simulink model "TestbedModel_v6"  (R2016a)
settings: Solver=ode23tb  StartTime=0.0  StopTime=20  RelTol=1e-3
undefined symbols (not defined in the file): K, Ki, Kp, magnitude, rev_comms_sink, tau
libraries: DAEMOT_Lib x4
(part 4 of 4)

== system TestbedModel_v6/Bus/Sink1 ==
  In1 : Inport
  tag scope: gdata_TestbedModel_v6BusSink1=global
  wires:
  In1/1 -> [gdata_TestbedModel_v6BusSink1]

== system TestbedModel_v6/Bus/Source1 ==
  Out1 : Outport
  wires:
  [gdata_TestbedModel_v6EffortSink9Sink1] -> Out1/1

== system TestbedModel_v6/Bus/Source2 ==
  Out1 : Outport
  wires:
  [gdata_TestbedModel_v6Converter2Sink1] -> Out1/1

== system TestbedModel_v6/Capacitor/Data_Sink ==
  " " : Inport
  tag scope: gdata_CapacitorData_Sink=global
  wires:
  " "/1 -> [gdata_CapacitorData_Sink]

== system TestbedModel_v6/Capacitor/Sink1 ==
  In1 : Inport
  tag scope: gdata_TestbedModel_v6CapacitorSink1=global
  wires:
  In1/1 -> [gdata_TestbedModel_v6CapacitorSink1]

== system TestbedModel_v6/Capacitor/Source1 ==
  Out1 : Outport
  wires:
  [gdata_TestbedModel_v6ResistorSink1] -> Out1/1

== system TestbedModel_v6/Capacitor1/Data_Sink ==
  " " : Inport
  tag scope: gdata_Capacitor1Data_Sink=global
  wires:
  " "/1 -> [gdata_Capacitor1Data_Sink]

== system TestbedModel_v6/Capacitor1/Sink1 ==
  In1 : Inport
  tag scope: gdata_TestbedModel_v6Capacitor1Sink1=global
  wires:
  In1/1 -> [gdata_TestbedModel_v6Capacitor1Sink1]

== system TestbedModel_v6/Capacitor1/Source1 ==
  Out1 : Outport
  wires:
  [gdata_TestbedModel_v6EffortSink13Sink1] -> Out1/1

== system TestbedModel_v6/Converter/Data_Sink ==
  " " : Inport
  tag scope: gdata_ConverterData_Sink=global
  wires:
  " "/1 -> [gdata_ConverterData_Sink]

== system TestbedModel_v6/Converter/Sink1 ==
  In1 : Inport
  tag scope: gdata_TestbedModel_v6ConverterSink1=global
  wires:
  In1/1 -> [gdata_TestbedModel_v6ConverterSink1]

== system TestbedModel_v6/Converter/Source1 ==
  Out1 : Outport
  wires:
  [gdata_TestbedModel_v6MotorSink1] -> Out1/1

== system TestbedModel_v6/Converter/Source2 ==
  Out1 : Outport
  wires:
  [gdata_TestbedModel_v6EffortSink2Sink1] -> Out1/1

== system TestbedModel_v6/Converter1/Data_Sink ==
  " " : Inport
  tag scope: gdata_Converter1Data_Sink=global
  wires:
  " "/1 -> [gdata_Converter1Data_Sink]

== system TestbedModel_v6/Converter1/Sink1 ==
  In1 : Inport
  tag scope: gdata_TestbedModel_v6Converter1Sink1=global
  wires:
  In1/1 -> [gdata_TestbedModel_v6Converter1Sink1]

== system TestbedModel_v6/Converter1/Source1 ==
  Out1 : Outport
  wires:
  [gdata_TestbedModel_v6InductorSink1] -> Out1/1

== system TestbedModel_v6/Converter1/Source2 ==
  Out1 : Outport
  wires:
  [gdata_TestbedModel_v6EffortSink5Sink1] -> Out1/1

== system TestbedModel_v6/Converter2/Data_Sink ==
  " " : Inport
  tag scope: gdata_Converter2Data_Sink=global
  wires:
  " "/1 -> [gdata_Converter2Data_Sink]

== system TestbedModel_v6/Converter2/Sink1 ==
  In1 : Inport
  tag scope: gdata_TestbedModel_v6Converter2Sink1=global
  wires:
  In1/1 -> [gdata_TestbedModel_v6Converter2Sink1]

== system TestbedModel_v6/Converter2/Source1 ==
  Out1 : Outport
  wires:
  [gdata_TestbedModel_v6Motor1Sink1] -> Out1/1

== system TestbedModel_v6/Converter2/Source2 ==
  Out1 : Outport
  wires:
  [gdata_TestbedModel_v6EffortSink8Sink1] -> Out1/1

== system TestbedModel_v6/Converter3/Data_Sink ==
  " " : Inport
  tag scope: gdata_Converter3Data_Sink=global
  wires:
  " "/1 -> [gdata_Converter3Data_Sink]

== system TestbedModel_v6/Converter3/Sink1 ==
  In1 : Inport
  tag scope: gdata_TestbedModel_v6Converter3Sink1=global
  wires:
  In1/1 -> [gdata_TestbedModel_v6Converter3Sink1]

== system TestbedModel_v6/Converter3/Source1 ==
  Out1 : Outport
  wires:
  [gdata_TestbedModel_v6Inductor1Sink1] -> Out1/1

== system TestbedModel_v6/Converter3/Source2 ==
  Out1 : Outport
  wires:
  [gdata_TestbedModel_v6EffortSink11Sink1] -> Out1/1

== system TestbedModel_v6/Data Manager/SubSystem1 ==
  Rename : Inport
  Bus : Outport
  wires:
  Rename/1 -> Bus/1

== system TestbedModel_v6/Data Manager1/SubSystem1 ==
  Rename : Inport
  Bus : Outport
  wires:
  Rename/1 -> Bus/1

== system TestbedModel_v6/Data Manager10/SubSystem1 ==
  Rename : Inport
  Bus : Outport
  wires:
  Rename/1 -> Bus/1

== system TestbedModel_v6/Data Manager11/SubSystem1 ==
  Rename : Inport
  Bus : Outport
  wires:
  Rename/1 -> Bus/1

== system TestbedModel_v6/Data Manager12/SubSystem1 ==
  Rename : Inport
  Bus : Outport
  wires:
  Rename/1 -> Bus/1

== system TestbedModel_v6/Data Manager13/SubSystem1 ==
  Rename : Inport
  Bus : Outport
  wires:
  Rename/1 -> Bus/1

== system TestbedModel_v6/Data Manager14/SubSystem1 ==
  Rename : Inport
  Bus : Outport
  wires:
  Rename/1 -> Bus/1

== system TestbedModel_v6/Data Manager15/SubSystem1 ==
  Rename : Inport
  Bus : Outport
  wires:
  Rename/1 -> Bus/1

== system TestbedModel_v6/Data Manager15/SubSystem2 ==
  Rename : Inport
  Bus : Outport
  wires:
  Rename/1 -> Bus/1

== system TestbedModel_v6/Data Manager16/SubSystem1 ==
  Rename : Inport
  Bus : Outport
  wires:
  Rename/1 -> Bus/1

== system TestbedModel_v6/Data Manager16/SubSystem2 ==
  Rename : Inport
  Bus : Outport
  wires:
  Rename/1 -> Bus/1

== system TestbedModel_v6/Data Manager16/SubSystem3 ==
  Rename : Inport
  Bus : Outport
  wires:
  Rename/1 -> Bus/1

== system TestbedModel_v6/Data Manager16/SubSystem4 ==
  Rename : Inport
  Bus : Outport
  wires:
  Rename/1 -> Bus/1

== system TestbedModel_v6/Data Manager17/SubSystem1 ==
  Rename : Inport
  Bus : Outport
  wires:
  Rename/1 -> Bus/1

== system TestbedModel_v6/Data Manager18/SubSystem1 ==
  Rename : Inport
  Bus : Outport
  wires:
  Rename/1 -> Bus/1

== system TestbedModel_v6/Data Manager19/SubSystem1 ==
  Rename : Inport
  Bus : Outport
  wires:
  Rename/1 -> Bus/1

== system TestbedModel_v6/Data Manager19/SubSystem2 ==
  Rename : Inport
  Bus : Outport
  wires:
  Rename/1 -> Bus/1

== system TestbedModel_v6/Data Manager2/SubSystem1 ==
  Rename : Inport
  Bus : Outport
  wires:
  Rename/1 -> Bus/1

== system TestbedModel_v6/Data Manager20/SubSystem1 ==
  Rename : Inport
  Bus : Outport
  wires:
  Rename/1 -> Bus/1

== system TestbedModel_v6/Data Manager21/SubSystem1 ==
  Rename : Inport
  Bus : Outport
  wires:
  Rename/1 -> Bus/1

== system TestbedModel_v6/Data Manager22/SubSystem1 ==
  Rename : Inport
  Bus : Outport
  wires:
  Rename/1 -> Bus/1

== system TestbedModel_v6/Data Manager23/SubSystem1 ==
  Rename : Inport
  Bus : Outport
  wires:
  Rename/1 -> Bus/1

== system TestbedModel_v6/Data Manager24/SubSystem1 ==
  Rename : Inport
  Bus : Outport
  wires:
  Rename/1 -> Bus/1

== system TestbedModel_v6/Data Manager25/SubSystem1 ==
  Rename : Inport
  Bus : Outport
  wires:
  Rename/1 -> Bus/1

== system TestbedModel_v6/Data Manager3/SubSystem1 ==
  Rename : Inport
  Bus : Outport
  wires:
  Rename/1 -> Bus/1

== system TestbedModel_v6/Data Manager4/SubSystem1 ==
  Rename : Inport
  Bus : Outport
  wires:
  Rename/1 -> Bus/1

== system TestbedModel_v6/Data Manager5/SubSystem1 ==
  Rename : Inport
  Bus : Outport
  wires:
  Rename/1 -> Bus/1

== system TestbedModel_v6/Data Manager6/SubSystem1 ==
  Rename : Inport
  Bus : Outport
  wires:
  Rename/1 -> Bus/1

== system TestbedModel_v6/Data Manager6/SubSystem2 ==
  Rename : Inport
  Bus : Outport
  wires:
  Rename/1 -> Bus/1

== system TestbedModel_v6/Data Manager7/SubSystem1 ==
  Rename : Inport
  Bus : Outport
  wires:
  Rename/1 -> Bus/1

== system TestbedModel_v6/Data Manager8/SubSystem1 ==
  Rename : Inport
  Bus : Outport
  wires:
  Rename/1 -> Bus/1

== system TestbedModel_v6/Data Manager9/SubSystem1 ==
  Rename : Inport
  Bus : Outport
  wires:
  Rename/1 -> Bus/1

== system TestbedModel_v6/Effort Sink1/Sink1 ==
  In1 : Inport
  tag scope: gdata_TestbedModel_v6EffortSink1Sink1=global
  wires:
  In1/1 -> [gdata_TestbedModel_v6EffortSink1Sink1]

== system TestbedModel_v6/Effort Sink10/Sink1 ==
  In1 : Inport
  tag scope: gdata_TestbedModel_v6EffortSink10Sink1=global
  wires:
  In1/1 -> [gdata_TestbedModel_v6EffortSink10Sink1]

== system TestbedModel_v6/Effort Sink11/Sink1 ==
  In1 : Inport
  tag scope: gdata_TestbedModel_v6EffortSink11Sink1=global
  wires:
  In1/1 -> [gdata_TestbedModel_v6EffortSink11Sink1]

== system TestbedModel_v6/Effort Sink12/Sink1 ==
  In1 : Inport
  tag scope: gdata_TestbedModel_v6EffortSink12Sink1=global
  wires:
  In1/1 -> [gdata_TestbedModel_v6EffortSink12Sink1]

== system TestbedModel_v6/Effort Sink13/Sink1 ==
  In1 : Inport
  tag scope: gdata_TestbedModel_v6EffortSink13Sink1=global
  wires:
  In1/1 -> [gdata_TestbedModel_v6EffortSink13Sink1]

== system TestbedModel_v6/Effort Sink14/Sink1 ==
  In1 : Inport
  tag scope: gdata_TestbedModel_v6EffortSink14Sink1=global
  wires:
  In1/1 -> [gdata_TestbedModel_v6EffortSink14Sink1]

== system TestbedModel_v6/Effort Sink15/Sink1 ==
  In1 : Inport
  tag scope: gdata_TestbedModel_v6EffortSink15Sink1=global
  wires:
  In1/1 -> [gdata_TestbedModel_v6EffortSink15Sink1]

== system TestbedModel_v6/Effort Sink16/Sink1 ==
  In1 : Inport
  tag scope: gdata_TestbedModel_v6EffortSink16Sink1=global
  wires:
  In1/1 -> [gdata_TestbedModel_v6EffortSink16Sink1]

== system TestbedModel_v6/Effort Sink2/Sink1 ==
  In1 : Inport
  tag scope: gdata_TestbedModel_v6EffortSink2Sink1=global
  wires:
  In1/1 -> [gdata_TestbedModel_v6EffortSink2Sink1]

== system TestbedModel_v6/Effort Sink3/Sink1 ==
  In1 : Inport
  tag scope: gdata_TestbedModel_v6EffortSink3Sink1=global
  wires:
  In1/1 -> [gdata_TestbedModel_v6EffortSink3Sink1]

== system TestbedModel_v6/Effort Sink4/Sink1 ==
  In1 : Inport
  tag scope: gdata_TestbedModel_v6EffortSink4Sink1=global
  wires:
  In1/1 -> [gdata_TestbedModel_v6EffortSink4Sink1]

== system TestbedModel_v6/Effort Sink5/Sink1 ==
  In1 : Inport
  tag scope: gdata_TestbedModel_v6EffortSink5Sink1=global
  wires:
  In1/1 -> [gdata_TestbedModel_v6EffortSink5Sink1]

== system TestbedModel_v6/Effort Sink6/Sink1 ==
  In1 : Inport
  tag scope: gdata_TestbedModel_v6EffortSink6Sink1=global
  wires:
  In1/1 -> [gdata_TestbedModel_v6EffortSink6Sink1]

== system TestbedModel_v6/Effort Sink7/Sink1 ==
  In1 : Inport
  tag scope: gdata_TestbedModel_v6EffortSink7Sink1=global
  wires:
  In1/1 -> [gdata_TestbedModel_v6EffortSink7Sink1]

== system TestbedModel_v6/Effort Sink8/Sink1 ==
  In1 : Inport
  tag scope: gdata_TestbedModel_v6EffortSink8Sink1=global
  wires:
  In1/1 -> [gdata_TestbedModel_v6EffortSink8Sink1]

== system TestbedModel_v6/Effort Sink9/Sink1 ==
  In1 : Inport
  tag scope: gdata_TestbedModel_v6EffortSink9Sink1=global
  wires:
  In1/1 -> [gdata_TestbedModel_v6EffortSink9Sink1]

== system TestbedModel_v6/Effort Source/Source1 ==
  Out1 : Outport
  wires:
  [gdata_TestbedModel_v6BatterySink1] -> Out1/1

== system TestbedModel_v6/Effort Source1/Source1 ==
  Out1 : Outport
  wires:
  [gdata_TestbedModel_v6VoltageBusSink1] -> Out1/1

== system TestbedModel_v6/Inductor/Data_Sink ==
  " " : Inport
  tag scope: gdata_InductorData_Sink=global
  wires:
  " "/1 -> [gdata_InductorData_Sink]

== system TestbedModel_v6/Inductor/Sink1 ==
  In1 : Inport
  tag scope: gdata_TestbedModel_v6InductorSink1=global
  wires:
  In1/1 -> [gdata_TestbedModel_v6InductorSink1]

== system TestbedModel_v6/Inductor/Source1 ==
  Out1 : Outport
  wires:
  [gdata_TestbedModel_v6CapacitorSink1] -> Out1/1

== system TestbedModel_v6/Inductor1/Data_Sink ==
  " " : Inport
  tag scope: gdata_Inductor1Data_Sink=global
  wires:
  " "/1 -> [gdata_Inductor1Data_Sink]

== system TestbedModel_v6/Inductor1/Sink1 ==
  In1 : Inport
  tag scope: gdata_TestbedModel_v6Inductor1Sink1=global
  wires:
  In1/1 -> [gdata_TestbedModel_v6Inductor1Sink1]

== system TestbedModel_v6/Inductor1/Source1 ==
  Out1 : Outport
  wires:
  [gdata_TestbedModel_v6Capacitor1Sink1] -> Out1/1

== system TestbedModel_v6/Motor/Data_Sink ==
  " " : Inport
  tag scope: gdata_MotorData_Sink=global
  wires:
  " "/1 -> [gdata_MotorData_Sink]

== system TestbedModel_v6/Motor/Sink1 ==
  In1 : Inport
  tag scope: gdata_TestbedModel_v6MotorSink1=global
  wires:
  In1/1 -> [gdata_TestbedModel_v6MotorSink1]

== system TestbedModel_v6/Motor/Source1 ==
  Out1 : Outport
  wires:
  [gdata_TestbedModel_v6EffortSink16Sink1] -> Out1/1

== system TestbedModel_v6/Motor/Source2 ==
  Out1 : Outport
  wires:
  [gdata_TestbedModel_v6EffortSink1Sink1] -> Out1/1

== system TestbedModel_v6/Motor1/Data_Sink ==
  " " : Inport
  tag scope: gdata_Motor1Data_Sink=global
  wires:
  " "/1 -> [gdata_Motor1Data_Sink]

== system TestbedModel_v6/Motor1/Sink1 ==
  In1 : Inport
  tag scope: gdata_TestbedModel_v6Motor1Sink1=global
  wires:
  In1/1 -> [gdata_TestbedModel_v6Motor1Sink1]

== system TestbedModel_v6/Motor1/Source1 ==
  Out1 : Outport
  wires:
  [gdata_TestbedModel_v6ShaftSink1] -> Out1/1

== system TestbedModel_v6/Motor1/Source2 ==
  Out1 : Outport
  wires:
  [gdata_TestbedModel_v6EffortSink7Sink1] -> Out1/1

== system TestbedModel_v6/Resistor/Data_Sink ==
  " " : Inport
  tag scope: gdata_ResistorData_Sink=global
  wires:
  " "/1 -> [gdata_ResistorData_Sink]

== system TestbedModel_v6/Resistor/Sink1 ==
  In1 : Inport
  tag scope: gdata_TestbedModel_v6ResistorSink1=global
  wires:
  In1/1 -> [gdata_TestbedModel_v6ResistorSink1]

== system TestbedModel_v6/Resistor/Source1 ==
  Out1 : Outport
  wires:
  [gdata_TestbedModel_v6EffortSink4Sink1] -> Out1/1

== system TestbedModel_v6/Resistor/Source2 ==
  Out1 : Outport
  wires:
  [gdata_TestbedModel_v6EffortSink3Sink1] -> Out1/1

== system TestbedModel_v6/Shaft/Data_Sink ==
  " " : Inport
  tag scope: gdata_ShaftData_Sink=global
  wires:
  " "/1 -> [gdata_ShaftData_Sink]

== system TestbedModel_v6/Shaft/Sink1 ==
  In1 : Inport
  tag scope: gdata_TestbedModel_v6ShaftSink1=global
  wires:
  In1/1 -> [gdata_TestbedModel_v6ShaftSink1]

== system TestbedModel_v6/Shaft/Source1 ==
  Out1 : Outport
  wires:
  [gdata_TestbedModel_v6AirVehicleSink1] -> Out1/1

== system TestbedModel_v6/Voltage Bus/Data_Sink ==
  " " : Inport
  tag scope: gdata_VoltageBusData_Sink=global
  wires:
  " "/1 -> [gdata_VoltageBusData_Sink]

== system TestbedModel_v6/Voltage Bus/Sink1 ==
  In1 : Inport
  tag scope: gdata_TestbedModel_v6VoltageBusSink1=global
  wires:
  In1/1 -> [gdata_TestbedModel_v6VoltageBusSink1]

== system TestbedModel_v6/Voltage Bus/Source1 ==
  Out1 : Outport
  wires:
  [gdata_TestbedModel_v6ConverterSink1] -> Out1/1

== system TestbedModel_v6/Voltage Bus/Source2 ==
  Out1 : Outport
  wires:
  [gdata_TestbedModel_v6Converter1Sink1] -> Out1/1

== matlab function TestbedModel_v6/Converter1/Current ==
  data: I_out input; D input; I_in output; s input; dir parameter
function I_in = current(I_out,D,s,dir)

if dir == 1 %Boost ===>
    if s == 0     % Buck Mode
        I_in = I_out/D;
    else    % Boost Mode
        I_in = I_out/(1-D);
    end
elseif dir == 2 %Boost <===
    if s == 0     % Buck Mode
        I_in = D*I_out;
    else    % Boost Mode
        I_in = (1-D)*I_out;
    end
end

== matlab function TestbedModel_v6/Converter1/Thermal ==
  data: Q input; T_dot output; Q_sink input; Cp parameter
function T_dot = Thermal(Q, Q_sink, Cp)
%% Load Temperature
T_dot = (1/Cp) * (Q - Q_sink);

== matlab function TestbedModel_v6/Converter1/Voltage ==
  data: V_in input; V_out output; I_in input; I_out input; D input; s input; V_D parameter; R_D parameter; R_s parameter; R_L parameter; Q output; dir parameter
function [V_out,Q]= voltage(V_in,I_in,I_out,D,s,V_D, R_D, R_s, R_L,dir)

if dir == 1 %Boost ===>
    I_L = I_in;
    if s == 0     % Buck Mode
        V_out = (1/D) * (V_in - R_L*I_L - D*R_s*I_L - (1-D)*R_D*I_L + (1-D)*V_D);
        Q = (1/D)^2 * (R_L*I_out^2 + D*R_s*I_out^2 + (1-D)*R_D*I_out^2);
    else    % Boost Mode
        V_out = (1/(1-D)) * (V_in - R_L*I_L - D*R_s*I_L - (1-D)*R_D*I_L - (1-D)*V_D);
        Q = (1/(1-D))^2 * (R_L*I_out^2 + D*R_s*I_out^2 + (1-D)*R_D*I_out^2);
    end
elseif dir == 2 %Boost <===
    I_L = I_out;
    if s == 0     % Buck Mode
        V_out = D*V_in - D*R_s*I_L - R_L*I_L - (1-D)*V_D - (1-D)*R_D*I_L;
        Q = (R_L*I_out^2 + D*R_s*I_out^2 + (1-D)*R_D*I_out^2);
    else    % Boost Mode
        V_out = (1-D)*V_in - D*R_s*I_L - R_L*I_L + (1-D)*V_D - (1-D)*R_D*I_L;
        Q = (R_L*I_out^2 + D*R_s*I_out^2 + (1-D)*R_D*I_out^2);
    end
end

== matlab function TestbedModel_v6/Inductor/Current ==
  data: V_in input; V_out input; dI_dt output; L parameter
function dI_dt = current(V_in, V_out,L)

dI_dt = (V_in-V_out)/L;

== matlab function TestbedModel_v6/Capacitor/Voltage ==
  data: I_in input; V_dot output; I_out input; C parameter
function V_dot = voltage(I_in, I_out,C)

V_dot = (1/C) * (I_in-I_out);

== matlab function TestbedModel_v6/Motor1/Current ==
  data: V_in input; I_in input; Kv parameter; R parameter; L parameter; omega input; dI_dt output; Q_elec output
function [dI_dt,Q_elec]= current(V_in,I_in,Kv, R, L,omega)


dI_dt = (1/L) * (V_in - R*I_in - Kv*omega);

Q_elec = R*I_in^2;

== matlab function TestbedModel_v6/Motor1/Thermal ==
  data: Q_elec input; Q_mech input; T_dot output; Q_sink input; Cp parameter
function T_dot = Thermal(Q_elec,Q_mech, Q_sink, Cp)
%% Load Temperature
T_dot = (1/Cp) * (Q_elec + Q_mech - Q_sink);

== matlab function TestbedModel_v6/Motor1/Torque ==
  data: I_in input; omega input; T_motor output; b parameter; c parameter; Q_mech output; Kv parameter
function [T_motor,Q_mech]= omega(I_in,omega, b,c,Kv)

T_motor = Kv*I_in - b*omega - c*(2./(1+exp(-5*omega)) - 1);

Q_mech = b*omega^2 + omega*(2./(1+exp(-5*omega)) - 1);

== matlab function TestbedModel_v6/Converter2/Current ==
  data: I_out input; D input; I_in output; s input; dir parameter
function I_in = current(I_out,D,s,dir)

if dir == 1 %Boost ===>
    if s == 0     % Buck Mode
        I_in = I_out/D;
    else    % Boost Mode
        I_in = I_out/(1-D);
    end
elseif dir == 2 %Boost <===
    if s == 0     % Buck Mode
        I_in = D*I_out;
    else    % Boost Mode
        I_in = (1-D)*I_out;
    end
end

== matlab function TestbedModel_v6/Converter2/Thermal ==
  data: Q input; T_dot output; Q_sink input; Cp parameter
function T_dot = Thermal(Q, Q_sink, Cp)
%% Load Temperature
T_dot = (1/Cp) * (Q - Q_sink);

== matlab function TestbedModel_v6/Converter2/Voltage ==
  data: V_in input; V_out output; I_in input; I_out input; D input; s input; V_D parameter; R_D parameter; R_s parameter; R_L parameter; Q output; dir parameter
function [V_out,Q]= voltage(V_in,I_in,I_out,D,s,V_D, R_D, R_s, R_L,dir)

if dir == 1 %Boost ===>
    I_L = I_in;
    if s == 0     % Buck Mode
        V_out = (1/D) * (V_in - R_L*I_L - D*R_s*I_L - (1-D)*R_D*I_L + (1-D)*V_D);
        Q = (1/D)^2 * (R_L*I_out^2 + D*R_s*I_out^2 + (1-D)*R_D*I_out^2);
    else    % Boost Mode
        V_out = (1/(1-D)) * (V_in - R_L*I_L - D*R_s*I_L - (1-D)*R_D*I_L - (1-D)*V_D);
        Q = (1/(1-D))^2 * (R_L*I_out^2 + D*R_s*I_out^2 + (1-D)*R_D*I_out^2);
    end
elseif dir == 2 %Boost <===
    I_L = I_out;
    if s == 0     % Buck Mode
        V_out = D*V_in - D*R_s*I_L - R_L*I_L - (1-D)*V_D - (1-D)*R_D*I_L;
        Q = (R_L*I_out^2 + D*R_s*I_out^2 + (1-D)*R_D*I_out^2);
    else    % Boost Mode
        V_out = (1-D)*V_in - D*R_s*I_L - R_L*I_L + (1-D)*V_D - (1-D)*R_D*I_L;
        Q = (R_L*I_out^2 + D*R_s*I_out^2 + (1-D)*R_D*I_out^2);
    end
end

== matlab function TestbedModel_v6/Converter3/Current ==
  data: I_out input; D input; I_in output; s input; dir parameter
function I_in = current(I_out,D,s,dir)

if dir == 1 %Boost ===>
    if s == 0     % Buck Mode
        I_in = I_out/D;
    else    % Boost Mode
        I_in = I_out/(1-D);
    end
elseif dir == 2 %Boost <===
    if s == 0     % Buck Mode
        I_in = D*I_out;
    else    % Boost Mode
        I_in = (1-D)*I_out;
    end
end

== matlab function TestbedModel_v6/Converter3/Thermal ==
  data: Q input; T_dot output; Q_sink input; Cp parameter
function T_dot = Thermal(Q, Q_sink, Cp)
%% Load Temperature
T_dot = (1/Cp) * (Q - Q_sink);

== matlab function TestbedModel_v6/Converter3/Voltage ==
  data: V_in input; V_out output; I_in input; I_out input; D input; s input; V_D parameter; R_D parameter; R_s parameter; R_L parameter; Q output; dir parameter
function [V_out,Q]= voltage(V_in,I_in,I_out,D,s,V_D, R_D, R_s, R_L,dir)

if dir == 1 %Boost ===>
    I_L = I_in;
    if s == 0     % Buck Mode
        V_out = (1/D) * (V_in - R_L*I_L - D*R_s*I_L - (1-D)*R_D*I_L + (1-D)*V_D);
        Q = (1/D)^2 * (R_L*I_out^2 + D*R_s*I_out^2 + (1-D)*R_D*I_out^2);
    else    % Boost Mode
        V_out = (1/(1-D)) * (V_in - R_L*I_L - D*R_s*I_L - (1-D)*R_D*I_L - (1-D)*V_D);
        Q = (1/(1-D))^2 * (R_L*I_out^2 + D*R_s*I_out^2 + (1-D)*R_D*I_out^2);
    end
elseif dir == 2 %Boost <===
    I_L = I_out;
    if s == 0     % Buck Mode
        V_out = D*V_in - D*R_s*I_L - R_L*I_L - (1-D)*V_D - (1-D)*R_D*I_L;
        Q = (R_L*I_out^2 + D*R_s*I_out^2 + (1-D)*R_D*I_out^2);
    else    % Boost Mode
        V_out = (1-D)*V_in - D*R_s*I_L - R_L*I_L + (1-D)*V_D - (1-D)*R_D*I_L;
        Q = (R_L*I_out^2 + D*R_s*I_out^2 + (1-D)*R_D*I_out^2);
    end
end

== matlab function TestbedModel_v6/Inductor1/Current ==
  data: V_in input; V_out input; dI_dt output; L parameter
function dI_dt = current(V_in, V_out,L)

dI_dt = (V_in-V_out)/L;

== matlab function TestbedModel_v6/Capacitor1/Voltage ==
  data: I_in input; V_dot output; I_out input; C parameter
function V_dot = voltage(I_in, I_out,C)

V_dot = (1/C) * (I_in-I_out);

== matlab function TestbedModel_v6/Battery/Electrical ==
  data: I input; V input; T_m input; V1_dot output; props input size=[1 7]; B_cap parameter; V2_dot output; SOC_dot output; V_T output; Q output; Np parameter; Ns parameter
function [V1_dot,V2_dot,SOC_dot,V_T,Q]= Electrical(I,V,T_m,props,B_cap, Np,Ns)
%% Electrical Effects Function
Rs = props(1)*Ns/Np;
R1 = props(2)*Ns/Np;
C1 = props(3)*Np/Ns;
R2 = props(4)*Ns/Np;
C2 = props(5)*Np/Ns;
dU_dt = props(6)*Ns;
V_ocv = props(7);
V1 = V(1);
V2 = V(2);
%outputs = zeros(1,5);

%% Voltage Dynamics
V1_dot = -V1/(R1*C1) + I/C1;
V2_dot = -V2/(R2*C2) + I/C2;

%% State of Charge Dynamic
SOC_dot = -I/(3600*B_cap*Np);

%% Terminal Voltage
V_T = V_ocv - V1 - V2 - I*Rs;

%% Heat Generation
Q_s = (T_m+273)*dU_dt/1000; %entropic heat
Q = I^2*Rs + V1^2/R1 + V2^2/R2 - I*Q_s/Np;

== matlab function TestbedModel_v6/Battery/Thermal ==
  data: Q input; Tc_dot output; T input; Q_sink input; C_c parameter; C_s parameter; R_cond parameter; Ts_dot output; Ns parameter; Np parameter
function [Tc_dot,Ts_dot]= Thermal(Q,T,Q_sink,C_c, C_s, R_cond, Ns, Np)
%% Thermal Effects Function
T_c = T(1);
T_s = T(2);

%% Core Temperature Dynamic
Tc_dot = (Q + Ns*Np*(T_s-T_c)/R_cond)/(Np*Ns*C_c);

%% Surface Temperature Dynamic
Ts_dot = (Ns*Np*(T_c-T_s)/R_cond - Q_sink)/(Np*Ns*C_s);

== matlab function TestbedModel_v6/Resistor/Electrical ==
  data: V_in input; out output; in input; R input; r_type parameter; Q output
function [out,Q]= voltage(V_in, in, R, r_type)
%% Output 

if r_type == 1 %voltage type
    out = (V_in - in)/R;
    Q = (V_in - in)/R^2;
else %current type
    out = V_in - in*R;
    Q = R^2*in;
end

== matlab function TestbedModel_v6/Resistor/Thermal ==
  data: Q input; T_dot output; Q_sink input; Cp parameter
function T_dot = Thermal(Q, Q_sink, Cp)
%% Load Temperature
T_dot = (1/Cp) * (Q - Q_sink);

== matlab function TestbedModel_v6/Motor/Current ==
  data: V_in input; I_in input; Kv parameter; R parameter; L parameter; omega input; dI_dt output; Q_elec output
function [dI_dt,Q_elec]= current(V_in,I_in,Kv, R, L,omega)


dI_dt = (1/L) * (V_in - R*I_in - Kv*omega);

Q_elec = R*I_in^2;

== matlab function TestbedModel_v6/Motor/Thermal ==
  data: Q_elec input; Q_mech input; T_dot output; Q_sink input; Cp parameter
function T_dot = Thermal(Q_elec,Q_mech, Q_sink, Cp)
%% Load Temperature
T_dot = (1/Cp) * (Q_elec + Q_mech - Q_sink);

== matlab function TestbedModel_v6/Motor/Torque ==
  data: I_in input; omega input; T_motor output; b parameter; c parameter; Q_mech output; Kv parameter
function [T_motor,Q_mech]= omega(I_in,omega, b,c,Kv)

T_motor = Kv*I_in - b*omega - c*(2./(1+exp(-5*omega)) - 1);

Q_mech = b*omega^2 + omega*(2./(1+exp(-5*omega)) - 1);

== matlab function TestbedModel_v6/Converter/Current ==
  data: I_out input; D input; I_in output; s input; dir parameter
function I_in = current(I_out,D,s,dir)

if dir == 1 %Boost ===>
    if s == 0     % Buck Mode
        I_in = I_out/D;
    else    % Boost Mode
        I_in = I_out/(1-D);
    end
elseif dir == 2 %Boost <===
    if s == 0     % Buck Mode
        I_in = D*I_out;
    else    % Boost Mode
        I_in = (1-D)*I_out;
    end
end

== matlab function TestbedModel_v6/Converter/Thermal ==
  data: Q input; T_dot output; Q_sink input; Cp parameter
function T_dot = Thermal(Q, Q_sink, Cp)
%% Load Temperature
T_dot = (1/Cp) * (Q - Q_sink);

== matlab function TestbedModel_v6/Converter/Voltage ==
  data: V_in input; V_out output; I_in input; I_out input; D input; s input; V_D parameter; R_D parameter; R_s parameter; R_L parameter; Q output; dir parameter
function [V_out,Q]= voltage(V_in,I_in,I_out,D,s,V_D, R_D, R_s, R_L,dir)

if dir == 1 %Boost ===>
    I_L = I_in;
    if s == 0     % Buck Mode
        V_out = (1/D) * (V_in - R_L*I_L - D*R_s*I_L - (1-D)*R_D*I_L + (1-D)*V_D);
        Q = (1/D)^2 * (R_L*I_out^2 + D*R_s*I_out^2 + (1-D)*R_D*I_out^2);
    else    % Boost Mode
        V_out = (1/(1-D)) * (V_in - R_L*I_L - D*R_s*I_L - (1-D)*R_D*I_L - (1-D)*V_D);
        Q = (1/(1-D))^2 * (R_L*I_out^2 + D*R_s*I_out^2 + (1-D)*R_D*I_out^2);
    end
elseif dir == 2 %Boost <===
    I_L = I_out;
    if s == 0     % Buck Mode
        V_out = D*V_in - D*R_s*I_L - R_L*I_L - (1-D)*V_D - (1-D)*R_D*I_L;
        Q = (R_L*I_out^2 + D*R_s*I_out^2 + (1-D)*R_D*I_out^2);
    else    % Boost Mode
        V_out = (1-D)*V_in - D*R_s*I_L - R_L*I_L + (1-D)*V_D - (1-D)*R_D*I_L;
        Q = (R_L*I_out^2 + D*R_s*I_out^2 + (1-D)*R_D*I_out^2);
    end
end

== matlab function TestbedModel_v6/Bus/current ==
  data: Iin_dot output; V_in input; V_out input; I_in input; I_out input; u_in input; u_out input; L parameter; R parameter; Iout_bar output
function [Iin_dot,Iout_bar]= current(V_in,V_out,I_in,I_out,u_in,u_out, L,R)
%% Input Current

Iin_dot = (1/L) * ((V_in - V_out).*u_in - I_in*R);
Iout_bar = u_out'*I_out;

== matlab function TestbedModel_v6/Bus/voltage ==
  data: I_in input; Ibar_out input; V_dot output; C parameter
function V_dot = voltage(I_in,Ibar_out,C)
%% Output Voltage

Ibar_in = sum(I_in);
V_dot = (Ibar_in - Ibar_out)/C;

== matlab function TestbedModel_v6/Shaft/current ==
  data: omega_dot output; tau_in input; tau_out input; J parameter
function omega_dot = speed(tau_in,tau_out,J)
%% Input Current

omega_dot = (1/J)*(sum(tau_in) - sum(tau_out));

== matlab function TestbedModel_v6/Air Vehicle/speed ==
  data: v input; omega input; props input; rho parameter; d parameter; v_dot output; tau output; M parameter; theta input; A parameter; C_D parameter; g parameter
function [v_dot,tau]= speed(v,omega, props,rho,d,M,theta,A, C_D,g)

C_T = props;

v_dot = (1/M)*((rho*d^4/(4*pi^2))*C_T*omega^2 - .5*rho*A*C_D*v^2 - M*g*sin(theta));
tau = (rho*d^4/(4*pi^2))*C_T*omega*v;


% dv_dt = (1/m) * (rho*(omega/(2*pi))^2*d^4*C_T - b*v);
% % tau = rho*(omega/(2*pi))^2*d^5*C_L*eta_prop;
% tau = v*omega*rho*(1/(2*pi))^2*d^4*C_T;

== matlab function TestbedModel_v6/Voltage Bus/current ==
  data: I_out input; u input; I_in output
function I_in = Current(I_out,u)
%% Input Current
I_in = u'*I_out;

%I_in = (V_in-V_out)/R_i;

== matlab function TestbedModel_v6/Voltage Bus/voltage ==
  data: V_in input; V_out output; u input
function V_out = Voltage(V_in,u)
%% Output Voltage

V_out = V_in.*u;

% if Gn == 1
%     V_dot = 0;
% else
%     V_dot = (I_in-sum(I_out))/G_cap;
% end
